simulink model "Real_Imag_Complex"  (R2020a)
settings: Solver=VariableStepAuto  StartTime=0.0  StopTime=10.0  RelTol=1e-3
settings Model: Creator=royde  LastModifiedBy=royde

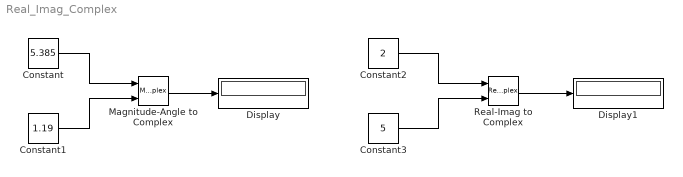
== system Real_Imag_Complex ==
  Constant : Constant  Value=5.385
  Constant1 : Constant  Value=1.19
  Constant2 : Constant  Value=2
  Constant3 : Constant  Value=5
  Display : Display
  Display1 : Display
  Magnitude-Angle to Complex : MagnitudeAngleToComplex
  Real-Imag to Complex : RealImagToComplex
  wires:
  Constant/1 -> Magnitude-Angle to Complex/1
  Constant1/1 -> Magnitude-Angle to Complex/2
  Magnitude-Angle to Complex/1 -> Display/1
  Constant2/1 -> Real-Imag to Complex/1
  Constant3/1 -> Real-Imag to Complex/2
  Real-Imag to Complex/1 -> Display1/1
